simulink model "tst_bus_outputasbus_combined"  (Simulink 8.0)
settings: Solver=ode45  StartTime=0.0  StopTime=10.0  RelTol=1e-3
settings Model: Creator=Marci  LastModifiedBy=Marci

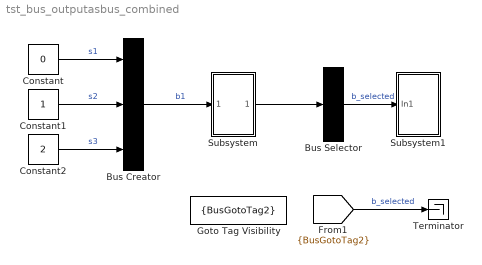
== system tst_bus_outputasbus_combined ==
  Bus Creator : BusCreator  Inputs=3
  Bus Selector : BusSelector  OutputSignals=s2,s3  OutputAsBus=on
  Constant : Constant  Value=0
  Constant1 : Constant
  Constant2 : Constant  Value=2
  Goto Tag Visibility : GotoTagVisibility  GotoTag=BusGotoTag2
  Subsystem : Subsystem
  Subsystem1 : Subsystem
  Terminator : Terminator
  wires:
  Constant/1 -> Bus Creator/1  "s1"
  Constant1/1 -> Bus Creator/2  "s2"
  Constant2/1 -> Bus Creator/3  "s3"
  [BusGotoTag2] -> Terminator/1  "b_selected"
  Bus Creator/1 -> Subsystem/1(In1)  "b1"
  Subsystem/1(Out1) -> Bus Selector/1
  Bus Selector/1 -> Subsystem1/1(In1)  "b_selected"

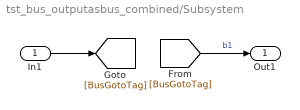
== system tst_bus_outputasbus_combined/Subsystem ==
  In1 : Inport
  Out1 : Outport
  wires:
  [BusGotoTag] -> Out1/1  "b1"
  In1/1 -> [BusGotoTag]

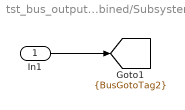
== system tst_bus_outputasbus_combined/Subsystem1 ==
  In1 : Inport
  tag scope: BusGotoTag2=scoped
  wires:
  In1/1 -> [BusGotoTag2]
